simulink model "Swarm_Robot_Base_2016b"  (R2016b)
settings: Solver=VariableStepAuto  StartTime=0.0  StopTime=20  FixedStep=0.1  RelTol=1e-3
values from neighbouring files (symbols this model uses):
  C = [25 8 1 0]    [Mech323Hw7.m]
settings Model: Creator=jfu1  LastModifiedBy=Shae

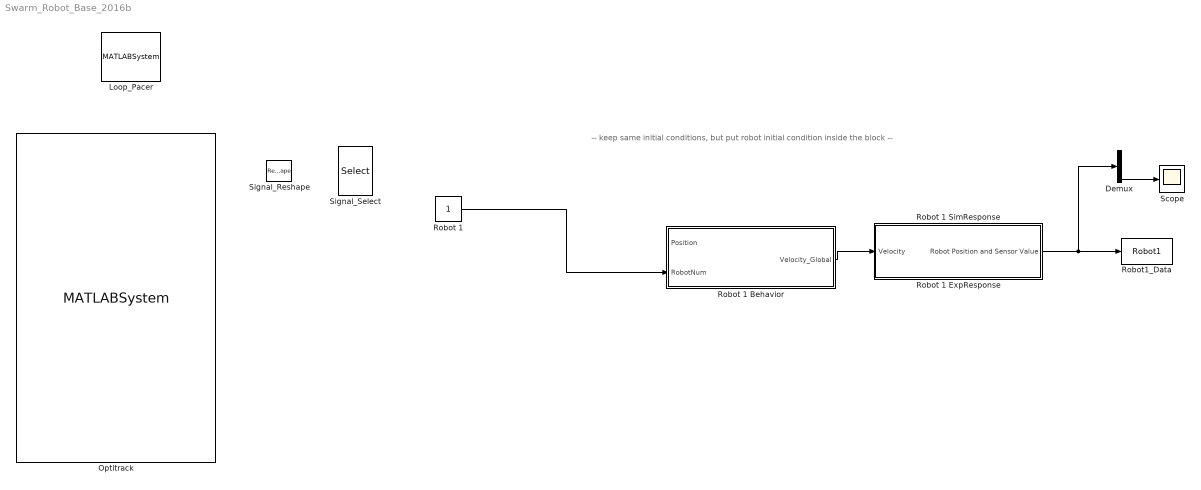
== system Swarm_Robot_Base_2016b ==
  note: -- keep same initial conditions, but put robot initial condition inside the block --
  Demux : Demux
  Loop_Pacer : MATLABSystem  System=LoopPacer  loopRate=0.1  debug=off
      mask Type: LoopPacer
      mask Display: disp('LoopPacer');
  Optitrack : MATLABSystem  System=OptiTrackRigidBody  coordinateTransformationMatrix=[ 1, 0, 0; 0, 0, 1; 0, -1, 0 ]  rigidBodyNames={}  orientationFormat=Euler angles  debug=on  natNetHostAddress=127.0.0.1  natNetClientAddress=127.0.0.1  dllPath=C:\DecaMATLAB\NatNetSDK\lib\x64\NatNetML.dll  unicast=off
      mask Type: OptiTrackRigidBody
      mask Display: disp('OptiTrackRigidBody');
  Robot 1 : Constant
  Robot 1 Behavior : Subsystem
  Robot 1 ExpResponse : Subsystem
  Robot 1 SimResponse : Subsystem
  Robot1_Data : ToWorkspace  VariableName=Robot1  SaveFormat=Timeseries  SampleTime=-1
  Scope : Scope
  Signal_Reshape : Reshape  OutputDimensions=6
  Signal_Select : Selector  InputPortWidth=6  IndexOptions=Index vector (dialog)  Indices=[1 2 6]  OutputSizes=1
  wires:
  Robot 1 SimResponse/1("Robot Position and Sensor Value ") -> Demux/1, Robot1_Data/1
  Robot 1 Behavior/1(Velocity_Global) -> Robot 1 SimResponse/1(Velocity)
  Demux/4 -> Scope/1
  Robot 1/1 -> Robot 1 Behavior/2(RobotNum)

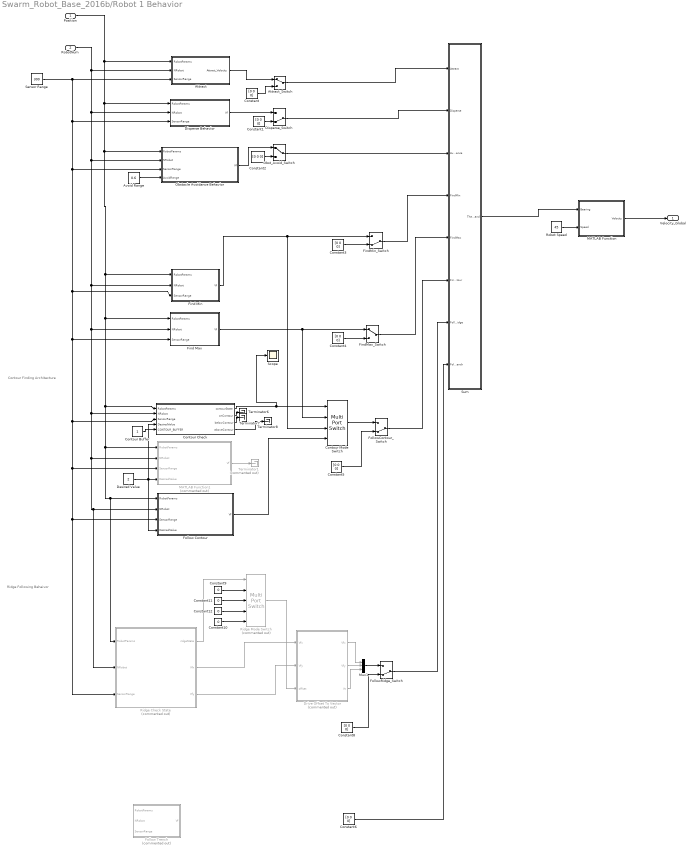
== system Swarm_Robot_Base_2016b/Robot 1 Behavior ==
  note: Contour Finding Architecture
  note: Ridge Following Behaivor
  Position : Inport
  RobotNum : Inport  Port=2
  Attract : MATLAB Function  TreatAsAtomicUnit=on
  Attract_Switch : ManualSwitch
  Avoid Range : Constant  Value=0.6
  Constant{,1..6,8} (8 alike) : Constant  Value=[0 0 0]
  Constant{9..12} (4 alike) : Constant  Value=0
  Contour Buffer : Constant
  Contour Check : MATLAB Function  TreatAsAtomicUnit=on
  Contour Mode Switch : MultiPortSwitch
  Desired Value : Constant  Value=2
  Disperse Behavior : MATLAB Function  TreatAsAtomicUnit=on
  Disperse_Switch : ManualSwitch  CurrentSetting=0
  Drive Offset To Vector : MATLAB Function  Commented=on  TreatAsAtomicUnit=on
  Find Max : MATLAB Function  TreatAsAtomicUnit=on
  Find Min : MATLAB Function  TreatAsAtomicUnit=on
  FindMax_Switch : ManualSwitch
  FindMin_Switch : ManualSwitch  CurrentSetting=0
  Follow Contour : MATLAB Function  TreatAsAtomicUnit=on
  Follow Trench : MATLAB Function  Commented=on  TreatAsAtomicUnit=on
  FollowContour_Switch : ManualSwitch  CurrentSetting=0
  FollowRidge_Switch : ManualSwitch  CurrentSetting=0
  MATLAB Function : MATLAB Function  TreatAsAtomicUnit=on
  MATLAB Function1 : MATLAB Function  Commented=on  TreatAsAtomicUnit=on
  Mux1 : Mux  Inputs=3
  Obst_Avoid_Switch : ManualSwitch
  Obstacle Avoidance Behavior : MATLAB Function  TreatAsAtomicUnit=on
  Ridge Check State : MATLAB Function  Commented=on  TreatAsAtomicUnit=on
  Ridge Mode Switch : MultiPortSwitch  Commented=on  Inputs=4
  Robot Speed : Constant  Value=45
  Scope : Scope
  Sensor Range : Constant  Value=300
  Sum : MATLAB Function  TreatAsAtomicUnit=on
  Terminator1 : Terminator  Commented=on
  Terminator6 : Terminator
  Terminator7 : Terminator
  Terminator8 : Terminator
  Velocity_Global : Outport
  wires:
  Robot Speed/1 -> MATLAB Function/2(Speed)
  Sum/1(ThetaCommand) -> MATLAB Function/1(Bearing)
  MATLAB Function/1(Velocity) -> Velocity_Global/1
  Constant8/1 -> FollowRidge_Switch/2
  Constant12/1 -> Ridge Mode Switch/4
  Constant5/1 -> FollowContour_Switch/2
  Ridge Check State/3(Vfy) -> Drive Offset To Vector/2("Vfy ")
  Ridge Check State/2(Vfx) -> Drive Offset To Vector/1("Vfx ")
  Ridge Check State/1(ridgeState) -> Ridge Mode Switch/1
  Obst_Avoid_Switch/1 -> Sum/3(Avoidance)
  Contour Check/2(onContour) -> Terminator6/1
  Constant4/1 -> FindMax_Switch/2
  Contour Check/1(contourState) -> Scope/1, Contour Mode Switch/1
  Sensor Range/1 -> Ridge Check State/3(SensorRange), Follow Contour/3(SensorRange), MATLAB Function1/3(SensorRange), Contour Check/3(SensorRange), Find Max/3(SensorRange), Find Min/3(SensorRange), Obstacle Avoidance Behavior/3(SensorRange), Disperse Behavior/3(SensorRange), Attract/3(SensorRange)
  Attract_Switch/1 -> Sum/1(Attract)
  Constant10/1 -> Ridge Mode Switch/5
  Find Max/1(Vf) -> FindMax_Switch/1, Contour Mode Switch/2
  Contour Check/3(belowContour) -> Terminator7/1
  Drive Offset To Vector/2(Vfy) -> Mux1/2
  RobotNum/1 -> Obstacle Avoidance Behavior/2(NRobot), Ridge Check State/2(NRobot), Follow Contour/2(NRobot), MATLAB Function1/2(NRobot), Contour Check/2(NRobot), Find Max/2(NRobot), Find Min/2(NRobot), Disperse Behavior/2(NRobot), Attract/2(NRobot)
  Disperse_Switch/1 -> Sum/2(Disperse)
  Mux1/1 -> FollowRidge_Switch/1
  Obstacle Avoidance Behavior/1(Vf) -> Obst_Avoid_Switch/1
  Constant1/1 -> Disperse_Switch/2
  MATLAB Function1/1(Vf) -> Terminator1/1
  Ridge Mode Switch/1 -> Drive Offset To Vector/3(offset)
  FindMin_Switch/1 -> Sum/4(FindMin)
  Contour Mode Switch/1 -> FollowContour_Switch/1
  Desired Value/1 -> Follow Contour/4(DesiredValue), Contour Check/4(DesiredValue), MATLAB Function1/4(DesiredValue)
  Disperse Behavior/1(Vf) -> Disperse_Switch/1
  Contour Check/4(aboveContour) -> Terminator8/1
  Constant11/1 -> Ridge Mode Switch/3
  Attract/1(Attract_Velocity) -> Attract_Switch/1
  Avoid Range/1 -> Obstacle Avoidance Behavior/4(AvoidRange)
  Constant/1 -> Attract_Switch/2
  Drive Offset To Vector/3(Vt) -> Mux1/3
  Constant9/1 -> Ridge Mode Switch/2
  Position/1 -> Ridge Check State/1(RobotParams), Follow Contour/1(RobotParams), MATLAB Function1/1(RobotParams), Contour Check/1(RobotParams), Find Max/1(RobotParams), Find Min/1(RobotParams), Obstacle Avoidance Behavior/1(RobotParams), Disperse Behavior/1(RobotParams), Attract/1(RobotParams)
  Drive Offset To Vector/1(Vfx) -> Mux1/1
  FollowContour_Switch/1 -> Sum/6(FindContour)
  Follow Contour/1(Vf) -> Contour Mode Switch/4
  Constant3/1 -> FindMin_Switch/2
  FindMax_Switch/1 -> Sum/5(FindMax)
  FollowRidge_Switch/1 -> Sum/7(FollowRidge)
  Find Min/1(Vf) -> FindMin_Switch/1, Contour Mode Switch/3
  Constant2/1 -> Obst_Avoid_Switch/2
  Constant6/1 -> Sum/8(FollowTrench)
  Contour Buffer/1 -> Contour Check/5(CONTOUR_BUFFER)

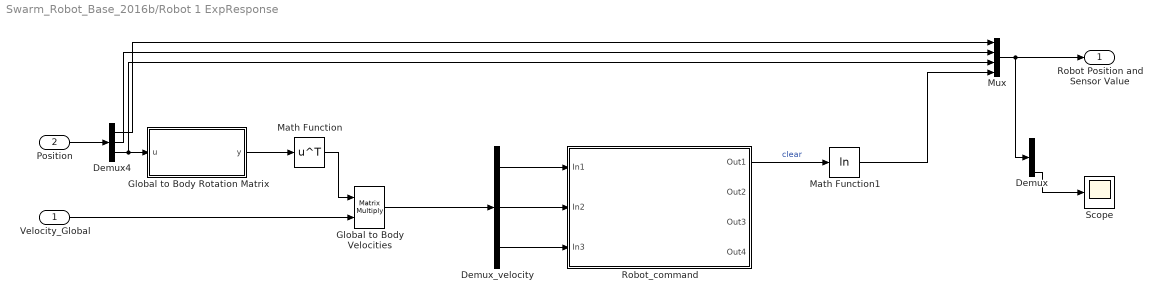
== system Swarm_Robot_Base_2016b/Robot 1 ExpResponse ==
  Velocity_Global : Inport
  Position : Inport  Port=2
  Demux : Demux
  Demux4 : Demux  Outputs=3
  Demux_velocity : Demux  Outputs=3
  Global to Body Velocities : Product  Multiplication=Matrix(*)
  Global to Body Rotation Matrix : MATLAB Function  TreatAsAtomicUnit=on
  Math Function : Math  Operator=transpose  SaturateOnIntegerOverflow=on
  Math Function1 : Math  Operator=log  SaturateOnIntegerOverflow=on
  Mux : Mux
  Robot_command : Subsystem  mask(DecabotMask){robotName=, decabotHelper=localhost, robotAddress=, useDataTurbine=off, useDirectSocket=on, debug=off}
      mask prompts: robotName "Robot name:"; decabotHelper "DecabotHelper/DataTurbine server:"; robotAddress "Robot network address (optional):"; useDataTurbine "Use DataTurbine"; useDirectSocket "Use direct robot TCP connection"; debug "Log debug messages"
      mask help: This is a masked subsystem that contains a Decabot block for bidirectional communication with a decabot over a direct TCP socket connection.
      mask init:
      | robotName = 'Nobody';
      | decabotHelper = 'localhost';
      | robotAddress = '';
      | useDataTurbine = true;
      | debug = true;
      mask TypeOptions robotName: decabot/robotName
      mask Callback robotName:
      | try
      |     set_param( gcb( ), 'Name', get_param( gcb( ), 'robotName' ) );
      | end
      mask TypeOptions decabotHelper: decabot/decabotHelper
      mask TypeOptions robotAddress: decabot/robotAddress
      mask TypeOptions useDataTurbine: decabot/useDataTurbine
      mask TypeOptions useDirectSocket: decabot/useDirectSocket
      mask TypeOptions debug: decabot/debug
      mask Display:
      | disp( [get_param( gcb( ), 'robotName' ) '\n\nDH: ' get_param( gcb( ), 'decabotHelper' ) ] );
      | 
      | port_label('input',1,'x_vel');
      | port_label('input',2,'y_vel');
      | port_label('input',3,'t_vel');
      | 
      | port_label('output',1,'clear');
      | port_label('output',2,'red');
      | port_label('output',3,'green');
      | port_label('output',4,'blue');
  Scope : Scope
  "Robot Position and Sensor Value " : Outport
  wires:
  Global to Body Velocities/1 -> Demux_velocity/1
  Velocity_Global/1 -> Global to Body Velocities/2
  Global to Body Rotation Matrix/1(y) -> Math Function/1
  Position/1 -> Demux4/1
  Math Function/1 -> Global to Body Velocities/1
  Demux4/3 -> Global to Body Rotation Matrix/1(u), Mux/3
  Demux_velocity/3 -> Robot_command/3(In3)
  Demux_velocity/1 -> Robot_command/1(In1)
  Robot_command/1(Out1) -> Math Function1/1  "clear"
  Demux_velocity/2 -> Robot_command/2(In2)
  Demux4/1 -> Mux/1
  Demux4/2 -> Mux/2
  Mux/1 -> Demux/1, "Robot Position and Sensor Value "/1
  Math Function1/1 -> Mux/4
  Demux/4 -> Scope/1

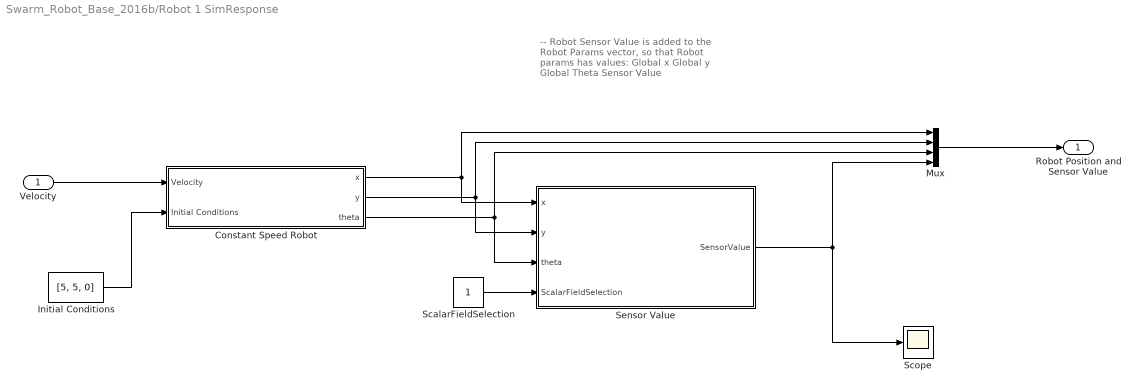
== system Swarm_Robot_Base_2016b/Robot 1 SimResponse ==
  note: -- Robot Sensor Value is added
      | to the Robot Params vector, so that
      | Robot params has values:
      |           Global x
      |           Global y
      |           Global Theta
      |           Sensor Value
  Velocity : Inport
  Constant Speed Robot : Subsystem
  Initial Conditions : Constant  Value=[5, 5, 0]
  Mux : Mux
  ScalarFieldSelection : Constant
  Scope : Scope
  Sensor Value : MATLAB Function  TreatAsAtomicUnit=on
  "Robot Position and Sensor Value " : Outport
  wires:
  Initial Conditions/1 -> Constant Speed Robot/2(Initial Conditions)
  Constant Speed Robot/1(x) -> Mux/1, Sensor Value/1(x)
  Velocity/1 -> Constant Speed Robot/1(Velocity)
  Mux/1 -> "Robot Position and Sensor Value "/1
  Sensor Value/1(SensorValue) -> Scope/1, Mux/4
  Constant Speed Robot/2(y) -> Mux/2, Sensor Value/2(y)
  Constant Speed Robot/3(theta) -> Mux/3, Sensor Value/3(theta)
  ScalarFieldSelection/1 -> Sensor Value/4(ScalarFieldSelection)

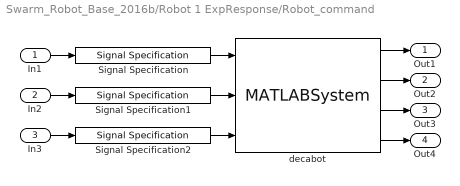
== system Swarm_Robot_Base_2016b/Robot 1 ExpResponse/Robot_command ==
  In1 : Inport
  In2 : Inport  Port=2
  In3 : Inport  Port=3
  Signal Specification : SignalSpecification  OutDataTypeStr=double  Dimensions=1
  Signal Specification1 : SignalSpecification  OutDataTypeStr=double  Dimensions=1
  Signal Specification2 : SignalSpecification  OutDataTypeStr=double  Dimensions=1
  decabot : MATLABSystem  System=Decabot  decabotHelper=localhost  useDataTurbine=off  useDirectSocket=on  debug=off
      mask Type: Decabot
      mask Display:
      | disp('\n\nDH: localhost');
      | port_label('input',1,'x_vel');
      | port_label('input',2,'y_vel');
      | port_label('input',3,'t_vel');
      | port_label('output',1,'clear');
      | port_label('output',2,'red');
      | port_label('output',3,'green');
      | port_label('output',4,'blue');
  Out1 : Outport
  Out2 : Outport  Port=2
  Out3 : Outport  Port=3
  Out4 : Outport  Port=4
  wires:
  Signal Specification2/1 -> decabot/3
  Signal Specification1/1 -> decabot/2
  Signal Specification/1 -> decabot/1
  In2/1 -> Signal Specification1/1
  decabot/4 -> Out4/1
  decabot/1 -> Out1/1
  decabot/3 -> Out3/1
  decabot/2 -> Out2/1
  In1/1 -> Signal Specification/1
  In3/1 -> Signal Specification2/1

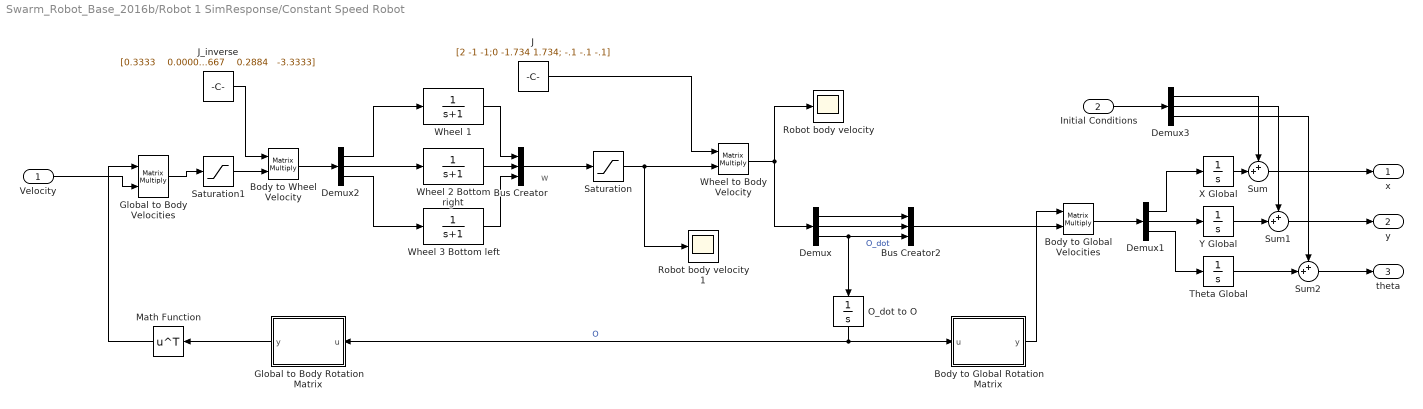
== system Swarm_Robot_Base_2016b/Robot 1 SimResponse/Constant Speed Robot ==
  note: w
  Velocity : Inport
  Initial Conditions : Inport  Port=2
  Body to Global Velocities : Product  Multiplication=Matrix(*)
  Body to Global Rotation Matrix : MATLAB Function  TreatAsAtomicUnit=on
  Body to Wheel Velocity : Product  Multiplication=Matrix(*)
  Bus Creator : BusCreator  Inputs=3
  Bus Creator2 : BusCreator  Inputs=3
  Demux{,1..3} (4 alike) : Demux  Outputs=3
  Global to Body Velocities : Product  Multiplication=Matrix(*)
  Global to Body Rotation Matrix : MATLAB Function  TreatAsAtomicUnit=on
  J : Constant  Value=[2 -1 -1;0 -1.734 1.734; -.1 -.1 -.1]
  J_inverse : Constant  Value=|
      | [0.3333    0.0000   -3.3333
      |  ;  -0.1667   -0.2884   -3.3333
      |  ;  -0.1667    0.2884   -3.3333]
  Math Function : Math  Operator=transpose  SaturateOnIntegerOverflow=on
  O_dot to O : Integrator
  "Robot body velocity " : Scope
  Robot body velocity 1 : Scope
  Saturation : Saturate  UpperLimit=6.28  LowerLimit=-6.28
  Saturation1 : Saturate  UpperLimit=2  LowerLimit=-2
  Sum : Sum  Inputs=++|
  Sum1 : Sum  Inputs=++|
  Sum2 : Sum  Inputs=++|
  Theta Global : Integrator
  Wheel 1 : TransferFcn  Denominator=[1 1]
  Wheel 2 Bottom right : TransferFcn  Denominator=[1 1]
  Wheel 3 Bottom left : TransferFcn  Denominator=[1 1]  ContinuousStateAttributes='orientation'
  Wheel to Body Velocity : Product  Multiplication=Matrix(*)
  X Global : Integrator
  Y Global : Integrator
  x : Outport
  y : Outport  Port=2
  theta : Outport  Port=3
  wires:
  Saturation/1 -> Robot body velocity 1/1, Wheel to Body Velocity/2
  Demux/1 -> Bus Creator2/1
  Demux2/1 -> Wheel 1/1
  Bus Creator/1 -> Saturation/1
  J_inverse/1 -> Body to Wheel Velocity/1
  Wheel to Body Velocity/1 -> Demux/1, "Robot body velocity "/1
  Bus Creator2/1 -> Body to Global Velocities/2
  Global to Body Velocities/1 -> Saturation1/1
  O_dot to O/1 -> Global to Body Rotation Matrix/1(u), Body to Global Rotation Matrix/1(u)  "O"
  Saturation1/1 -> Body to Wheel Velocity/2
  Body to Wheel Velocity/1 -> Demux2/1
  Wheel 1/1 -> Bus Creator/1
  Demux2/2 -> Wheel 2 Bottom right/1
  J/1 -> Wheel to Body Velocity/1
  Body to Global Rotation Matrix/1(y) -> Body to Global Velocities/1
  Demux/3 -> O_dot to O/1, Bus Creator2/3  "O_dot"
  Wheel 3 Bottom left/1 -> Bus Creator/3
  Demux2/3 -> Wheel 3 Bottom left/1
  Demux/2 -> Bus Creator2/2
  Wheel 2 Bottom right/1 -> Bus Creator/2
  Body to Global Velocities/1 -> Demux1/1
  Demux1/1 -> X Global/1
  Demux1/2 -> Y Global/1
  X Global/1 -> Sum/2
  Y Global/1 -> Sum1/2
  Demux1/3 -> Theta Global/1
  Initial Conditions/1 -> Demux3/1
  Demux3/1 -> Sum/1
  Sum/1 -> x/1
  Demux3/2 -> Sum1/1
  Theta Global/1 -> Sum2/2
  Demux3/3 -> Sum2/1
  Sum2/1 -> theta/1
  Sum1/1 -> y/1
  Velocity/1 -> Global to Body Velocities/2
  Global to Body Rotation Matrix/1(y) -> Math Function/1
  Math Function/1 -> Global to Body Velocities/1

== matlab function Swarm_Robot_Base_2016b/Robot 1 Behavior/Contour Check ==
  data: contourState output; RobotParams input; NRobot input; SensorRange input; DesiredValue input; onContour output; belowContour output; aboveContour output; CONTOUR_BUFFER input
function [contourState, onContour, belowContour, aboveContour] = ContourCheck(RobotParams, NRobot, SensorRange,  DesiredValue,CONTOUR_BUFFER)
% calls the SwarmSimOnContour behavior function

[contourState, onContour, belowContour, aboveContour] = SwarmSimOnContour(RobotParams, NRobot, SensorRange, DesiredValue,CONTOUR_BUFFER);

end

== matlab function Swarm_Robot_Base_2016b/Robot 1 Behavior/Find Max ==
  data: RobotParams input; Vf output; NRobot input; SensorRange input
function Vf = FindMax(RobotParams, NRobot, SensorRange)
% calls the SwarmSimFindMax behavior

Vf= SwarmSimFindMax(RobotParams, NRobot, SensorRange);
end

== matlab function Swarm_Robot_Base_2016b/Robot 1 Behavior/Follow Contour ==
  data: RobotParams input; Vf output; NRobot input; SensorRange input; DesiredValue input
 function Vf  = FollowContour(RobotParams, NRobot, SensorRange,  DesiredValue)
% calls the SwarmSimFollow behavior

[Vf] = SwarmSimFollowContour(RobotParams, NRobot, SensorRange, DesiredValue);

end

== matlab function Swarm_Robot_Base_2016b/Robot 1 ExpResponse/Global to Body Rotation Matrix ==
  data: u input; y output
function y = fcn(u)

y = [cos(u) -sin(u) 0; sin(u) cos(u) 0; 0 0 1];

%y= [cos(u) sin(u) 0; -sin(u) cos(u) 0; 0 0 1]; 

% y= A';

== matlab function Swarm_Robot_Base_2016b/Robot 1 Behavior/Follow Trench ==
  data: RobotParams input; Vf output; NRobot input; SensorRange input
function Vf = FollowTrench(RobotParams, NRobot, SensorRange)
% Matlab Function block calls the SwarmSimFindMin function 

Vf= SwarmSimFollowTrench(RobotParams, NRobot,SensorRange); 

end

== matlab function Swarm_Robot_Base_2016b/Robot 1 Behavior/Drive Offset To Vector ==
  data: Vfx output size=[1 3] [-100000000000..10000000000]; Vfx input; Vfy input; offset input; Vfy output; Vt output
function [Vfx,Vfy,Vt]    = DriveOffsetToVector(Vfx, Vfy, offset)
% Matlab Function block calls the .....

[Vfx,Vfy,Vt] = SwarmSimDriveOffsetToVector(Vfx, Vfy, offset); 

end

== matlab function Swarm_Robot_Base_2016b/Robot 1 Behavior/MATLAB Function1 ==
  data: RobotParams input; Vf output; NRobot input; SensorRange input; DesiredValue input
function Vf   = Contour_Finding(RobotParams, NRobot, SensorRange, DesiredValue)

[Vf]  = SwarmSimFindContour(RobotParams, NRobot, SensorRange, DesiredValue);

end

== matlab function Swarm_Robot_Base_2016b/Robot 1 Behavior/Ridge Check State ==
  data: ridgeState output size=1 [0..5]; RobotParams input; NRobot input; SensorRange input; Vfx output size=1; Vfy output size=1
function [ridgeState, Vfx, Vfy] = RidgeCheckState(RobotParams, NRobot, SensorRange)
% calls the SwarmSimRidgeCheck behavior function

[ridgeState, Vfx, Vfy] = SwarmSimRidgeCheck(RobotParams, NRobot, SensorRange);

end

== matlab function Swarm_Robot_Base_2016b/Robot 1 Behavior/Disperse Behavior ==
  data: Vf output; RobotParams input; NRobot input; SensorRange input
function Vf = disperse(RobotParams,NRobot,SensorRange)
Vf= SwarmSimDisperse(RobotParams, NRobot, SensorRange);
end

== matlab function Swarm_Robot_Base_2016b/Robot 1 Behavior/Obstacle Avoidance Behavior ==
  data: Vf output; RobotParams input; NRobot input; SensorRange input; AvoidRange input
 function Vf = ObstacleAvoidance(RobotParams,NRobot, SensorRange, AvoidRange)

% This Matlab Function block calls the SwarmSimObstacleAvoid function. For
% details on function, see SwarmSimObstacleAvoid.m

[Vf] = SwarmSimObstacleAvoid(RobotParams, NRobot, SensorRange, AvoidRange); 
end

== matlab function Swarm_Robot_Base_2016b/Robot 1 SimResponse/Sensor Value ==
  data: x input; SensorValue output; y input; theta input; ScalarFieldSelection input
function SensorValue = SensorValue_from_position(x, y, theta,ScalarFieldSelection)
% this function determines the Sensor Value for the given robot for the
% desired concentration profile
 %%%%%%%%%%%%%%%%%%%%%%%%%%%%%%%%
 
 %NEED TO UPDATE TO CALL A FUNCTION 
 
 % from the 1x3 vector CurrentPosition, extract current global (x,y) and
 
 %note that in most applications theta will be unused

% given the current x,y position, determine the Sensor Value based off
% current (x,y) position

%To change the concentration profile, change here:

%concentration= sqrt(x^2 + y^2); %simple source function centered at origin
SensorValue=0;
SensorValue= readScalarField(x,y,ScalarFieldSelection);

end

== matlab function Swarm_Robot_Base_2016b/Robot 1 Behavior/Find Min ==
  data: RobotParams input; Vf output; NRobot input; SensorRange input
function Vf = FindMin(RobotParams, NRobot, SensorRange)
% Matlab Function block calls the SwarmSimFindMin function 

Vf= SwarmSimFindMin(RobotParams, NRobot,SensorRange); 
end

== matlab function Swarm_Robot_Base_2016b/Robot 1 Behavior/Attract ==
  data: RobotParams input; Attract_Velocity output; NRobot input; SensorRange input
function Attract_Velocity = Attract(RobotParams, NRobot, SensorRange)
%calls the SwarmSimAttract function to determine robot velocities for
%attract behavior. 

Attract_Velocity = SwarmSimAttract(RobotParams,NRobot,SensorRange);

== matlab function Swarm_Robot_Base_2016b/Robot 1 Behavior/Sum ==
  data: Attract input; ThetaCommand output; Disperse input; Avoidance input; FindMin input; FindMax input; FindContour input; FollowRidge input; FollowTrench input
function ThetaCommand = VelocitySum(Attract,Disperse,Avoidance,FindMin,FindMax,FindContour,FollowRidge,FollowTrench)

% This Matlab Function block calls the SwarmSimSum function. For details on
% SwarmSimSum function, see SwarmSimSum.m

ThetaCommand = SwarmSimSum(Attract, Disperse, Avoidance, FindMin, FindMax, FindContour, FollowRidge, FollowTrench);

end

== matlab function Swarm_Robot_Base_2016b/Robot 1 SimResponse/Constant Speed Robot/Body to Global Rotation Matrix ==
  data: u input; y output
function y = fcn(u)

y = [cos(u) -sin(u) 0; sin(u) cos(u) 0; 0 0 1];

== matlab function Swarm_Robot_Base_2016b/Robot 1 SimResponse/Constant Speed Robot/Global to Body Rotation Matrix ==
  data: u input; y output
function y = fcn(u)

y = [cos(u) -sin(u) 0; sin(u) cos(u) 0; 0 0 1];

%y= [cos(u) sin(u) 0; -sin(u) cos(u) 0; 0 0 1]; 

% y= A';

== matlab function Swarm_Robot_Base_2016b/Robot 1 Behavior/MATLAB Function ==
  data: Bearing input; Speed input; Velocity output
function Velocity = rob_vel_from_bearing(Bearing, Speed)
% function block calculates robot velocity based off user-set constant
% robot velocity and bearing calculated from behaviors.

if Bearing == NaN;
    Vx= 0 ;
    Vy= 0;
    Vt= 0;
else
    Vx= Speed*cos(Bearing);
    Vy= Speed*sin(Bearing);
    Vt= 0.0;
end

Velocity = [Vx ; Vy ; Vt];
end
